simulink model "Proyecto_final_sim_pert_R2020a"  (R2020a)
settings: Solver=VariableStepAuto  StartTime=0.0  StopTime=10.0  RelTol=1e-3
values from neighbouring files (symbols this model uses):
  A = [0 0 1 0 ... (first row only)    [main.m]
  B = [0;0;(Kg*Ki*n_total)/(Rm*(Jb+mb*delta_2^2)*((L/d)));0]    [main.m]
  C = [0 1 0 0]    [main.m]
  D = 0    [main.m]
  L = 0.425    [main.m]    (also in mylqr.m = L'; pole_placement.m = L1)
undefined symbols (not defined in the file or in its folder): K_itae, K_lqr, K_pole, Kext_itae, Kext_lqr, Kext_pole, Kp_itae, Kp_lqr, Kp_pole, rank, sysob_cl_itae, sysob_cl_lqr, sysob_cl_pole, sysob_itae, sysob_lqr, sysob_pole, sysobext_itae, sysobext_lqr, sysobext_pole
settings Model: Creator=Windows_10  LastModifiedBy=sergi

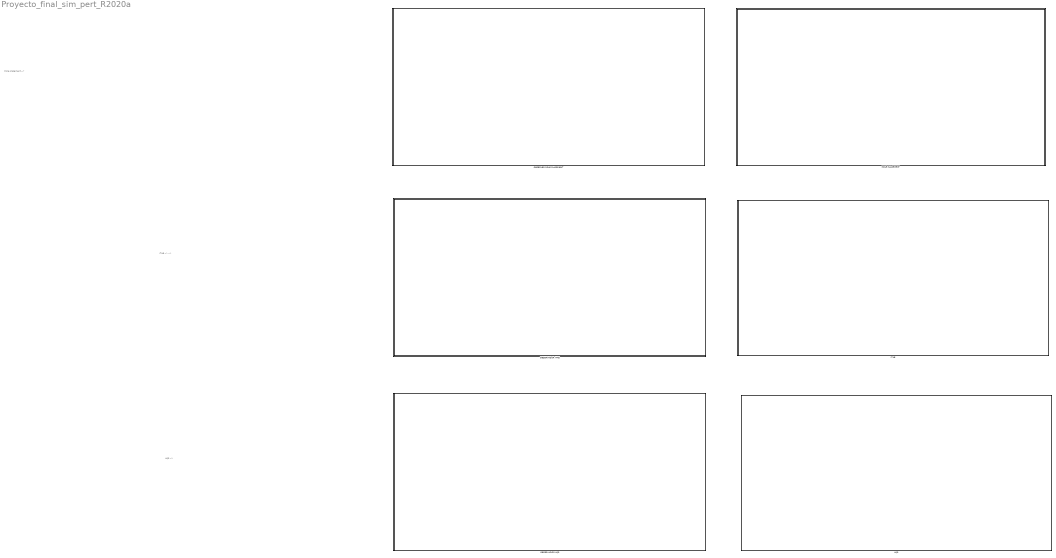
== system Proyecto_final_sim_pert_R2020a ==
  note: LQR -->
  note: ITAE --> -->
  note: Pole placement -->
  ITAE : Subsystem
  LQR : Subsystem
  OBSERVADOR ITAE : Subsystem
  OBSERVADOR LQR : Subsystem
  "OBSERVER POLE PLACEMENT " : Subsystem
  POLE PLACEMENT : Subsystem

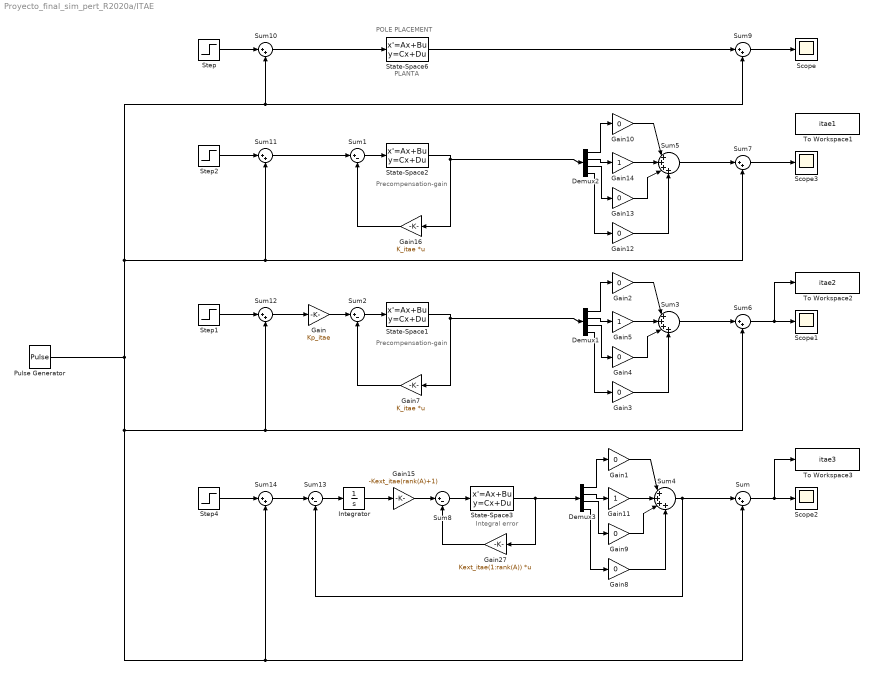
== system Proyecto_final_sim_pert_R2020a/ITAE ==
  note: POLE PLACEMENT
  note: PLANTA
  note: Precompensation-gain
  note: Precompensation-gain
  note: Integral error
  Demux1 : Demux
  Demux2 : Demux
  Demux3 : Demux
  Gain : Gain  Gain=Kp_itae
  Gain{1..4,8..10,12..13} (9 alike) : Gain  Gain=0
  Gain11 : Gain
  Gain14 : Gain
  Gain15 : Gain  Gain=-Kext_itae(rank(A)+1)
  Gain16 : Gain  Gain=K_itae  Multiplication=Matrix(K*u)
  Gain27 : Gain  Gain=Kext_itae(1:rank(A))  Multiplication=Matrix(K*u)
  Gain5 : Gain
  Gain7 : Gain  Gain=K_itae  Multiplication=Matrix(K*u)
  Integrator : Integrator
  Pulse Generator : DiscretePulseGenerator  PulseType=Time based  Period=10  PulseWidth=5
  Scope{,1..3} (4 alike) : Scope
  State-Space{1..3,6} (4 alike) : StateSpace  A=A  B=B  C=eye(rank(A))  D=zeros(rank(A),1)  InitialCondition=0
  Step{,1..2,4} (4 alike) : Step  Time=0  After=L/2  SampleTime=0
  Sum{,6..7,9..12,14} (8 alike) : Sum  Inputs=|++
  Sum{1..2,8,13} (4 alike) : Sum  Inputs=|+-
  Sum3 : Sum  Inputs=|++++
  Sum4 : Sum  Inputs=|++++
  Sum5 : Sum  Inputs=|++++
  To Workspace1 : ToWorkspace  VariableName=itae1  SaveFormat=Timeseries  SampleTime=-1
  To Workspace2 : ToWorkspace  VariableName=itae2  SaveFormat=Timeseries  SampleTime=-1
  To Workspace3 : ToWorkspace  VariableName=itae3  SaveFormat=Timeseries  SampleTime=-1
  wires:
  Sum2/1 -> State-Space1/1
  Gain/1 -> Sum2/1
  Gain7/1 -> Sum2/2
  Gain5/1 -> Sum3/2
  Demux1/1 -> Gain2/1
  Demux1/4 -> Gain3/1
  Gain2/1 -> Sum3/1
  Demux1/3 -> Gain4/1
  Gain4/1 -> Sum3/3
  Demux1/2 -> Gain5/1
  State-Space1/1 -> Demux1/1, Gain7/1
  Gain3/1 -> Sum3/4
  Demux2/3 -> Gain13/1
  Gain10/1 -> Sum5/1
  Demux2/4 -> Gain12/1
  Gain14/1 -> Sum5/2
  Demux2/2 -> Gain14/1
  Gain12/1 -> Sum5/4
  Gain16/1 -> Sum1/2
  State-Space2/1 -> Demux2/1, Gain16/1
  Gain13/1 -> Sum5/3
  Sum1/1 -> State-Space2/1
  Demux2/1 -> Gain10/1
  Gain8/1 -> Sum4/4
  Demux3/3 -> Gain9/1
  Sum8/1 -> State-Space3/1
  Gain1/1 -> Sum4/1
  Gain11/1 -> Sum4/2
  Demux3/2 -> Gain11/1
  Gain9/1 -> Sum4/3
  Demux3/1 -> Gain1/1
  Gain15/1 -> Sum8/1
  Demux3/4 -> Gain8/1
  Sum13/1 -> Integrator/1
  Gain27/1 -> Sum8/2
  Sum4/1 -> Sum/1, Sum13/2
  Integrator/1 -> Gain15/1
  State-Space3/1 -> Gain27/1, Demux3/1
  Sum/1 -> To Workspace3/1, Scope2/1
  Sum3/1 -> Sum6/1
  Sum6/1 -> To Workspace2/1, Scope1/1
  Sum5/1 -> Sum7/1
  Sum7/1 -> Scope3/1
  Sum9/1 -> Scope/1
  State-Space6/1 -> Sum9/1
  Step/1 -> Sum10/1
  Sum10/1 -> State-Space6/1
  Step2/1 -> Sum11/1
  Sum11/1 -> Sum1/1
  Step1/1 -> Sum12/1
  Sum12/1 -> Gain/1
  Sum14/1 -> Sum13/1
  Step4/1 -> Sum14/1
  Pulse Generator/1 -> Sum11/2, Sum7/2, Sum10/2, Sum9/2, Sum6/2, Sum12/2, Sum/2, Sum14/2

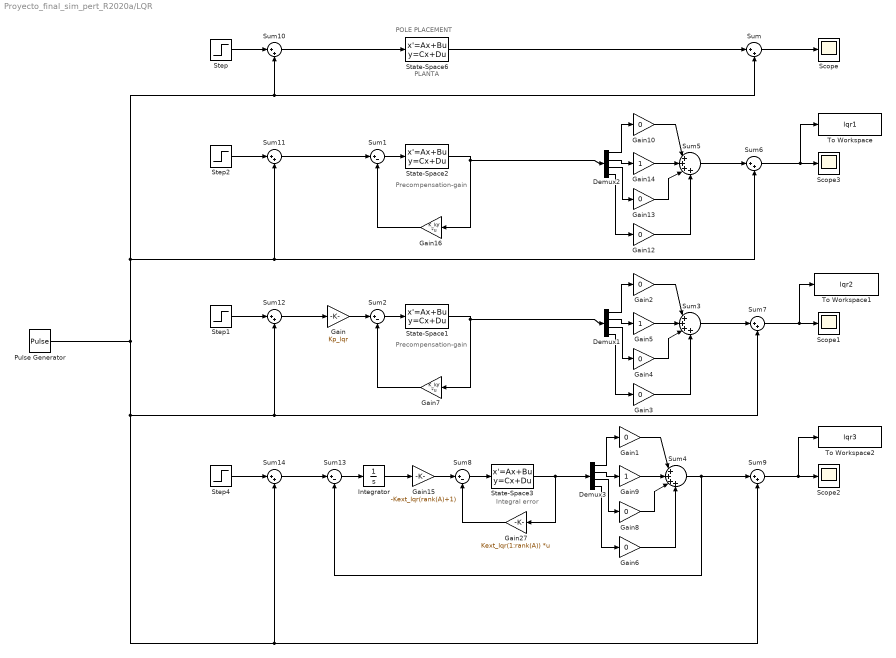
== system Proyecto_final_sim_pert_R2020a/LQR ==
  note: POLE PLACEMENT
  note: PLANTA
  note: Precompensation-gain
  note: Precompensation-gain
  note: Integral error
  Demux1 : Demux
  Demux2 : Demux
  Demux3 : Demux
  Gain : Gain  Gain=Kp_lqr
  Gain{1..4,6,8,10,12..13} (9 alike) : Gain  Gain=0
  Gain14 : Gain
  Gain15 : Gain  Gain=-Kext_lqr(rank(A)+1)
  Gain16 : Gain  Gain=K_lqr  Multiplication=Matrix(K*u)
  Gain27 : Gain  Gain=Kext_lqr(1:rank(A))  Multiplication=Matrix(K*u)
  Gain5 : Gain
  Gain7 : Gain  Gain=K_lqr  Multiplication=Matrix(K*u)
  Gain9 : Gain
  Integrator : Integrator
  Pulse Generator : DiscretePulseGenerator  PulseType=Time based  Period=10  PulseWidth=5
  Scope{,1..3} (4 alike) : Scope
  State-Space{1..3,6} (4 alike) : StateSpace  A=A  B=B  C=eye(rank(A))  D=zeros(rank(A),1)  InitialCondition=0
  Step{,1..2,4} (4 alike) : Step  Time=0  After=L/2  SampleTime=0
  Sum{,6..7,9..12,14} (8 alike) : Sum  Inputs=|++
  Sum{1..2,8,13} (4 alike) : Sum  Inputs=|+-
  Sum3 : Sum  Inputs=|++++
  Sum4 : Sum  Inputs=|++++
  Sum5 : Sum  Inputs=|++++
  To Workspace : ToWorkspace  VariableName=lqr1  SaveFormat=Timeseries  SampleTime=-1
  To Workspace1 : ToWorkspace  VariableName=lqr2  SaveFormat=Timeseries  SampleTime=-1
  To Workspace2 : ToWorkspace  VariableName=lqr3  SaveFormat=Timeseries  SampleTime=-1
  wires:
  Sum2/1 -> State-Space1/1
  Gain/1 -> Sum2/1
  Gain7/1 -> Sum2/2
  Gain5/1 -> Sum3/2
  Demux1/1 -> Gain2/1
  Demux1/4 -> Gain3/1
  Gain2/1 -> Sum3/1
  Demux1/3 -> Gain4/1
  Gain4/1 -> Sum3/3
  Demux1/2 -> Gain5/1
  State-Space1/1 -> Demux1/1, Gain7/1
  Gain3/1 -> Sum3/4
  Demux2/3 -> Gain13/1
  Gain10/1 -> Sum5/1
  Demux2/4 -> Gain12/1
  Gain14/1 -> Sum5/2
  Demux2/2 -> Gain14/1
  Gain12/1 -> Sum5/4
  Gain16/1 -> Sum1/2
  State-Space2/1 -> Demux2/1, Gain16/1
  Gain13/1 -> Sum5/3
  Sum1/1 -> State-Space2/1
  Demux2/1 -> Gain10/1
  Gain15/1 -> Sum8/1
  Sum13/1 -> Integrator/1
  Gain27/1 -> Sum8/2
  State-Space3/1 -> Demux3/1, Gain27/1
  Integrator/1 -> Gain15/1
  Sum8/1 -> State-Space3/1
  Gain6/1 -> Sum4/4
  Gain8/1 -> Sum4/3
  Demux3/3 -> Gain8/1
  Demux3/2 -> Gain9/1
  Demux3/1 -> Gain1/1
  Demux3/4 -> Gain6/1
  Gain1/1 -> Sum4/1
  Gain9/1 -> Sum4/2
  Sum4/1 -> Sum13/2, Sum9/1
  Sum9/1 -> To Workspace2/1, Scope2/1
  Sum7/1 -> To Workspace1/1, Scope1/1
  Sum6/1 -> To Workspace/1, Scope3/1
  Sum5/1 -> Sum6/1
  Sum/1 -> Scope/1
  State-Space6/1 -> Sum/1
  Step/1 -> Sum10/1
  Step2/1 -> Sum11/1
  Step1/1 -> Sum12/1
  Step4/1 -> Sum14/1
  Sum10/1 -> State-Space6/1
  Sum11/1 -> Sum1/1
  Sum12/1 -> Gain/1
  Sum14/1 -> Sum13/1
  Sum3/1 -> Sum7/1
  Pulse Generator/1 -> Sum11/2, Sum6/2, Sum10/2, Sum/2, Sum14/2, Sum9/2, Sum12/2, Sum7/2

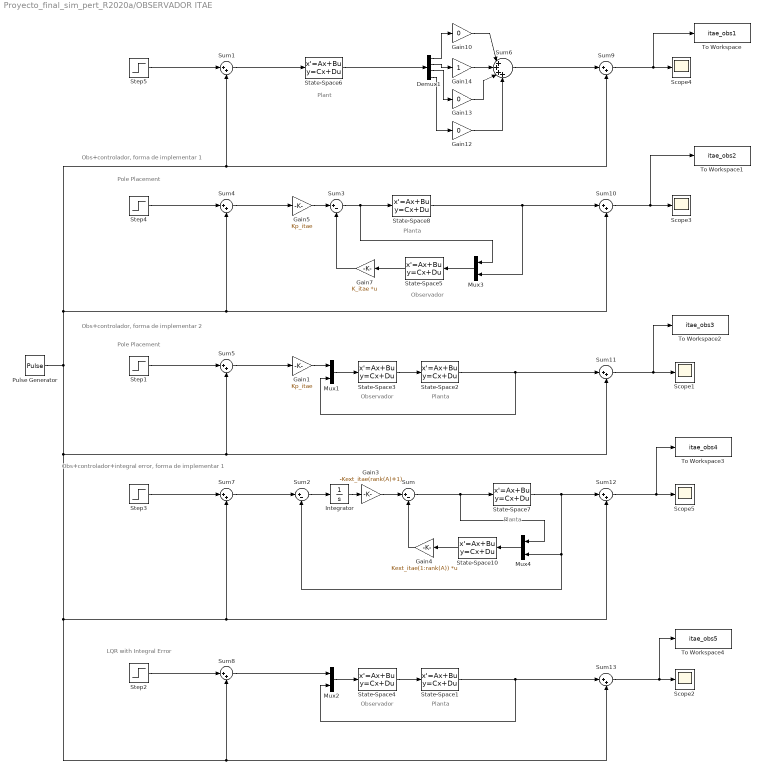
== system Proyecto_final_sim_pert_R2020a/OBSERVADOR ITAE ==
  note: Planta
  note: Planta
  note: Plant
  note: Observador
  note: Pole Placement
  note: Observador
  note: Pole Placement
  note: Obs+controlador, forma de implementar 1
  note: Obs+controlador, forma de implementar 2
  note: Observador
  note: Planta
  note: LQR with Integral Error
  note: Obs+controlador+integral error, forma de implementar 1
  note: Planta
  Demux1 : Demux
  Gain1 : Gain  Gain=Kp_itae
  Gain10 : Gain  Gain=0
  Gain12 : Gain  Gain=0
  Gain13 : Gain  Gain=0
  Gain14 : Gain
  Gain3 : Gain  Gain=-Kext_itae(rank(A)+1)
  Gain4 : Gain  Gain=Kext_itae(1:rank(A))  Multiplication=Matrix(K*u)
  Gain5 : Gain  Gain=Kp_itae
  Gain7 : Gain  Gain=K_itae  Multiplication=Matrix(K*u)
  Integrator : Integrator
  Mux{1..4} (4 alike) : Mux  Inputs=2
  Pulse Generator : DiscretePulseGenerator  PulseType=Time based  Period=10  PulseWidth=5
  Scope{1..5} (5 alike) : Scope
  State-Space{1..2,7..8} (4 alike) : StateSpace  A=A  B=B  C=C  D=D  InitialCondition=0
  State-Space10 : StateSpace  A=sysob_itae.A  B=sysob_itae.B  C=sysob_itae.C  D=sysob_itae.D  InitialCondition=0
  State-Space3 : StateSpace  A=sysob_cl_itae.A  B=sysob_cl_itae.B  C=sysob_cl_itae.C  D=sysob_cl_itae.D  InitialCondition=0
  State-Space4 : StateSpace  A=sysobext_itae.A  B=sysobext_itae.B  C=sysobext_itae.C  D=sysobext_itae.D  InitialCondition=0
  State-Space5 : StateSpace  A=sysob_itae.A  B=sysob_itae.B  C=sysob_itae.C  D=sysob_itae.D  InitialCondition=0
  State-Space6 : StateSpace  A=A  B=B  C=eye(rank(A))  D=zeros(rank(A),1)  InitialCondition=0
  Step{1..5} (5 alike) : Step  Time=0  After=L/2  SampleTime=0
  Sum : Sum  Inputs=|+-
  Sum{1,4..5,7..13} (10 alike) : Sum  Inputs=|++
  Sum2 : Sum  Inputs=|+-
  Sum3 : Sum  Inputs=|+-
  Sum6 : Sum  Inputs=|++++
  To Workspace : ToWorkspace  VariableName=itae_obs1  SaveFormat=Timeseries  SampleTime=-1
  To Workspace1 : ToWorkspace  VariableName=itae_obs2  SaveFormat=Timeseries  SampleTime=-1
  To Workspace2 : ToWorkspace  VariableName=itae_obs3  SaveFormat=Timeseries  SampleTime=-1
  To Workspace3 : ToWorkspace  VariableName=itae_obs4  SaveFormat=Timeseries  SampleTime=-1
  To Workspace4 : ToWorkspace  VariableName=itae_obs5  SaveFormat=Timeseries  SampleTime=-1
  wires:
  Gain7/1 -> Sum3/2
  State-Space2/1 -> Mux1/2, Sum11/1
  Demux1/2 -> Gain14/1
  State-Space3/1 -> State-Space2/1
  Demux1/3 -> Gain13/1
  Gain1/1 -> Mux1/1
  Gain13/1 -> Sum6/3
  Mux1/1 -> State-Space3/1
  State-Space5/1 -> Gain7/1
  Gain5/1 -> Sum3/1
  Mux3/1 -> State-Space5/1
  Sum3/1 -> Mux3/1, State-Space8/1
  State-Space8/1 -> Sum10/1, Mux3/2
  Demux1/1 -> Gain10/1
  State-Space6/1 -> Demux1/1
  Gain10/1 -> Sum6/1
  Gain14/1 -> Sum6/2
  Demux1/4 -> Gain12/1
  Gain12/1 -> Sum6/4
  Mux2/1 -> State-Space4/1
  State-Space1/1 -> Sum13/1, Mux2/2
  State-Space4/1 -> State-Space1/1
  Integrator/1 -> Gain3/1
  Gain3/1 -> Sum/1
  Mux4/1 -> State-Space10/1
  State-Space10/1 -> Gain4/1
  Sum2/1 -> Integrator/1
  Sum/1 -> State-Space7/1, Mux4/1
  Gain4/1 -> Sum/2
  State-Space7/1 -> Sum12/1, Sum2/2, Mux4/2
  Step5/1 -> Sum1/1
  Sum1/1 -> State-Space6/1
  Step4/1 -> Sum4/1
  Sum4/1 -> Gain5/1
  Step1/1 -> Sum5/1
  Sum5/1 -> Gain1/1
  Step3/1 -> Sum7/1
  Sum7/1 -> Sum2/1
  Step2/1 -> Sum8/1
  Sum8/1 -> Mux2/1
  Sum6/1 -> Sum9/1
  Sum9/1 -> To Workspace/1, Scope4/1
  Sum10/1 -> To Workspace1/1, Scope3/1
  Sum11/1 -> To Workspace2/1, Scope1/1
  Sum12/1 -> To Workspace3/1, Scope5/1
  Sum13/1 -> To Workspace4/1, Scope2/1
  Pulse Generator/1 -> Sum4/2, Sum10/2, Sum1/2, Sum9/2, Sum5/2, Sum11/2, Sum7/2, Sum12/2, Sum8/2, Sum13/2

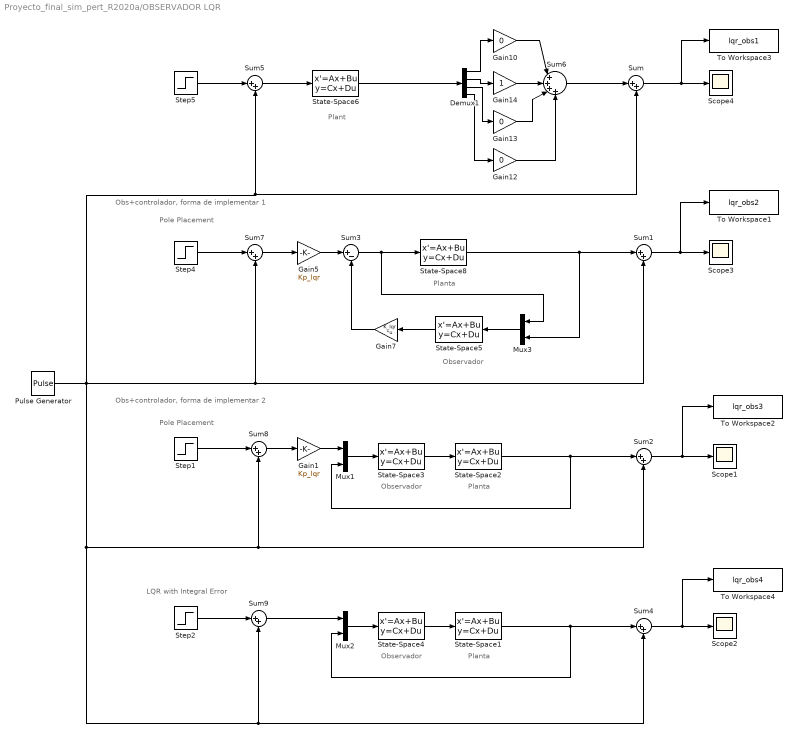
== system Proyecto_final_sim_pert_R2020a/OBSERVADOR LQR ==
  note: Planta
  note: Planta
  note: Plant
  note: Observador
  note: Pole Placement
  note: Observador
  note: Pole Placement
  note: Obs+controlador, forma de implementar 1
  note: Obs+controlador, forma de implementar 2
  note: Observador
  note: Planta
  note: LQR with Integral Error
  Demux1 : Demux
  Gain1 : Gain  Gain=Kp_lqr
  Gain10 : Gain  Gain=0
  Gain12 : Gain  Gain=0
  Gain13 : Gain  Gain=0
  Gain14 : Gain
  Gain5 : Gain  Gain=Kp_lqr
  Gain7 : Gain  Gain=K_lqr  Multiplication=Matrix(K*u)
  Mux1 : Mux  Inputs=2
  Mux2 : Mux  Inputs=2
  Mux3 : Mux  Inputs=2
  Pulse Generator : DiscretePulseGenerator  PulseType=Time based  Period=10  PulseWidth=5
  Scope{1..4} (4 alike) : Scope
  State-Space1 : StateSpace  A=A  B=B  C=C  D=D  InitialCondition=0
  State-Space2 : StateSpace  A=A  B=B  C=C  D=D  InitialCondition=0
  State-Space3 : StateSpace  A=sysob_cl_lqr.A  B=sysob_cl_lqr.B  C=sysob_cl_lqr.C  D=sysob_cl_lqr.D  InitialCondition=0
  State-Space4 : StateSpace  A=sysobext_lqr.A  B=sysobext_lqr.B  C=sysobext_lqr.C  D=sysobext_lqr.D  InitialCondition=0
  State-Space5 : StateSpace  A=sysob_lqr.A  B=sysob_lqr.B  C=sysob_lqr.C  D=sysob_lqr.D  InitialCondition=0
  State-Space6 : StateSpace  A=A  B=B  C=eye(rank(A))  D=zeros(rank(A),1)  InitialCondition=0
  State-Space8 : StateSpace  A=A  B=B  C=C  D=D  InitialCondition=0
  Step{1..2,4..5} (4 alike) : Step  Time=0  After=L/2  SampleTime=0
  Sum{,1..2,4..5,7..9} (8 alike) : Sum  Inputs=|++
  Sum3 : Sum  Inputs=|+-
  Sum6 : Sum  Inputs=|++++
  To Workspace1 : ToWorkspace  VariableName=lqr_obs2  SaveFormat=Timeseries  SampleTime=-1
  To Workspace2 : ToWorkspace  VariableName=lqr_obs3  SaveFormat=Timeseries  SampleTime=-1
  To Workspace3 : ToWorkspace  VariableName=lqr_obs1  SaveFormat=Timeseries  SampleTime=-1
  To Workspace4 : ToWorkspace  VariableName=lqr_obs4  SaveFormat=Timeseries  SampleTime=-1
  wires:
  Gain7/1 -> Sum3/2
  State-Space2/1 -> Sum2/1, Mux1/2
  Demux1/2 -> Gain14/1
  State-Space3/1 -> State-Space2/1
  Demux1/3 -> Gain13/1
  Gain1/1 -> Mux1/1
  Gain13/1 -> Sum6/3
  Mux1/1 -> State-Space3/1
  State-Space5/1 -> Gain7/1
  Gain5/1 -> Sum3/1
  Mux3/1 -> State-Space5/1
  Sum3/1 -> Mux3/1, State-Space8/1
  State-Space8/1 -> Sum1/1, Mux3/2
  Demux1/1 -> Gain10/1
  State-Space6/1 -> Demux1/1
  Gain10/1 -> Sum6/1
  Gain14/1 -> Sum6/2
  Demux1/4 -> Gain12/1
  Gain12/1 -> Sum6/4
  Mux2/1 -> State-Space4/1
  State-Space1/1 -> Sum4/1, Mux2/2
  State-Space4/1 -> State-Space1/1
  Sum6/1 -> Sum/1
  Sum/1 -> To Workspace3/1, Scope4/1
  Sum1/1 -> Scope3/1, To Workspace1/1
  Sum2/1 -> Scope1/1, To Workspace2/1
  Sum4/1 -> Scope2/1, To Workspace4/1
  Sum5/1 -> State-Space6/1
  Step5/1 -> Sum5/1
  Sum7/1 -> Gain5/1
  Step4/1 -> Sum7/1
  Sum8/1 -> Gain1/1
  Step1/1 -> Sum8/1
  Sum9/1 -> Mux2/1
  Step2/1 -> Sum9/1
  Pulse Generator/1 -> Sum1/2, Sum7/2, Sum8/2, Sum2/2, Sum4/2, Sum9/2, Sum/2, Sum5/2

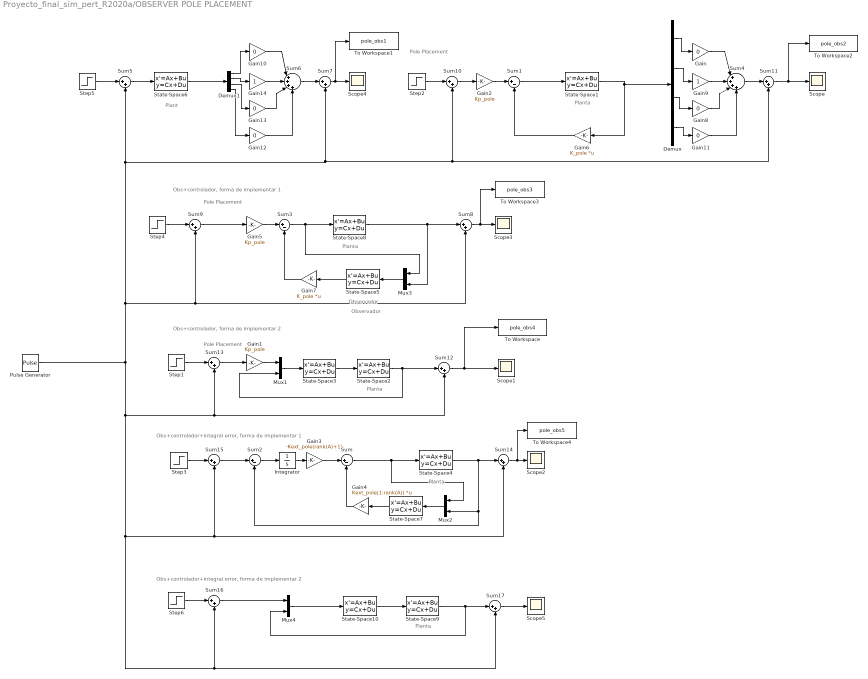
== system Proyecto_final_sim_pert_R2020a/OBSERVER POLE PLACEMENT  ==
  note: Planta
  note: Planta
  note: Planta
  note: Planta
  note: Planta
  note: Plant
  note: Obs+controlador+integral error, forma de implementar 1
  note: Observador
  note: Pole Placement
  note: Pole Placement
  note: Observador
  note: Pole Placement
  note: Obs+controlador, forma de implementar 1
  note: Obs+controlador, forma de implementar 2
  note: Obs+controlador+integral error, forma de implementar 2
  Demux : Demux
  Demux1 : Demux
  Gain{,8,10..13} (6 alike) : Gain  Gain=0
  Gain1 : Gain  Gain=Kp_pole
  Gain14 : Gain
  Gain2 : Gain  Gain=Kp_pole
  Gain3 : Gain  Gain=-Kext_pole(rank(A)+1)
  Gain4 : Gain  Gain=Kext_pole(1:rank(A))  Multiplication=Matrix(K*u)
  Gain5 : Gain  Gain=Kp_pole
  Gain6 : Gain  Gain=K_pole  Multiplication=Matrix(K*u)
  Gain7 : Gain  Gain=K_pole  Multiplication=Matrix(K*u)
  Gain9 : Gain
  Integrator : Integrator
  Mux{1..4} (4 alike) : Mux  Inputs=2
  Pulse Generator : DiscretePulseGenerator  PulseType=Time based  Period=10  PulseWidth=5
  Scope{,1..5} (6 alike) : Scope
  State-Space1 : StateSpace  A=A  B=B  C=eye(rank(A))  D=zeros(rank(A),1)  InitialCondition=0
  State-Space10 : StateSpace  A=sysobext_pole.A  B=sysobext_pole.B  C=sysobext_pole.C  D=sysobext_pole.D  InitialCondition=0
  State-Space{2,4,8..9} (4 alike) : StateSpace  A=A  B=B  C=C  D=D  InitialCondition=0
  State-Space3 : StateSpace  A=sysob_cl_pole.A  B=sysob_cl_pole.B  C=sysob_cl_pole.C  D=sysob_cl_pole.D  InitialCondition=0
  State-Space5 : StateSpace  A=sysob_pole.A  B=sysob_pole.B  C=sysob_pole.C  D=sysob_pole.D  InitialCondition=0
  State-Space6 : StateSpace  A=A  B=B  C=eye(rank(A))  D=zeros(rank(A),1)  InitialCondition=0
  State-Space7 : StateSpace  A=sysob_pole.A  B=sysob_pole.B  C=sysob_pole.C  D=sysob_pole.D  InitialCondition=0
  Step{1..6} (6 alike) : Step  Time=0  After=L/2  SampleTime=0
  Sum{,1..3} (4 alike) : Sum  Inputs=|+-
  Sum{5,7..17} (12 alike) : Sum  Inputs=|++
  Sum4 : Sum  Inputs=|++++
  Sum6 : Sum  Inputs=|++++
  To Workspace : ToWorkspace  VariableName=pole_obs4  SaveFormat=Timeseries  SampleTime=-1
  To Workspace1 : ToWorkspace  VariableName=pole_obs1  SaveFormat=Timeseries  SampleTime=-1
  To Workspace2 : ToWorkspace  VariableName=pole_obs2  SaveFormat=Timeseries  SampleTime=-1
  To Workspace3 : ToWorkspace  VariableName=pole_obs3  SaveFormat=Timeseries  SampleTime=-1
  To Workspace4 : ToWorkspace  VariableName=pole_obs5  SaveFormat=Timeseries  SampleTime=-1
  wires:
  Gain4/1 -> Sum/2
  Gain7/1 -> Sum3/2
  Gain6/1 -> Sum1/2
  Sum/1 -> State-Space4/1, Mux2/1
  Demux1/2 -> Gain14/1
  State-Space3/1 -> State-Space2/1
  Demux1/3 -> Gain13/1
  Demux/2 -> Gain9/1
  Gain1/1 -> Mux1/1
  Gain13/1 -> Sum6/3
  Mux1/1 -> State-Space3/1
  State-Space5/1 -> Gain7/1
  Gain5/1 -> Sum3/1
  Sum1/1 -> State-Space1/1
  State-Space4/1 -> Sum14/1, Sum2/2, Mux2/2
  Mux3/1 -> State-Space5/1
  Sum3/1 -> Mux3/1, State-Space8/1
  Gain2/1 -> Sum1/1
  State-Space8/1 -> Sum8/1, Mux3/2
  Mux4/1 -> State-Space10/1
  Demux/1 -> Gain/1
  Mux2/1 -> State-Space7/1
  State-Space7/1 -> Gain4/1
  Gain/1 -> Sum4/1
  Demux1/1 -> Gain10/1
  Sum2/1 -> Integrator/1
  State-Space6/1 -> Demux1/1
  Gain10/1 -> Sum6/1
  Gain3/1 -> Sum/1
  Integrator/1 -> Gain3/1
  State-Space1/1 -> Demux/1, Gain6/1
  State-Space9/1 -> Sum17/1, Mux4/2
  Gain8/1 -> Sum4/3
  Gain14/1 -> Sum6/2
  Gain9/1 -> Sum4/2
  Demux/3 -> Gain8/1
  State-Space10/1 -> State-Space9/1
  Demux/4 -> Gain11/1
  Gain11/1 -> Sum4/4
  Demux1/4 -> Gain12/1
  Gain12/1 -> Sum6/4
  Step5/1 -> Sum5/1
  Sum6/1 -> Sum7/1
  Sum7/1 -> To Workspace1/1, Scope4/1
  Sum8/1 -> To Workspace3/1, Scope3/1
  Sum5/1 -> State-Space6/1
  Pulse Generator/1 -> Sum10/2, Sum11/2, Sum7/2, Sum5/2, Sum9/2, Sum8/2, Sum12/2, Sum13/2, Sum17/2, Sum16/2, Sum15/2, Sum14/2
  Step4/1 -> Sum9/1
  Sum9/1 -> Gain5/1
  Sum4/1 -> Sum11/1
  Sum11/1 -> To Workspace2/1, Scope/1
  Step2/1 -> Sum10/1
  Sum10/1 -> Gain2/1
  Sum12/1 -> To Workspace/1, Scope1/1
  Sum13/1 -> Gain1/1
  Step1/1 -> Sum13/1
  State-Space2/1 -> Sum12/1, Mux1/2
  Sum14/1 -> To Workspace4/1, Scope2/1
  Sum15/1 -> Sum2/1
  Step3/1 -> Sum15/1
  Step6/1 -> Sum16/1
  Sum16/1 -> Mux4/1
  Sum17/1 -> Scope5/1

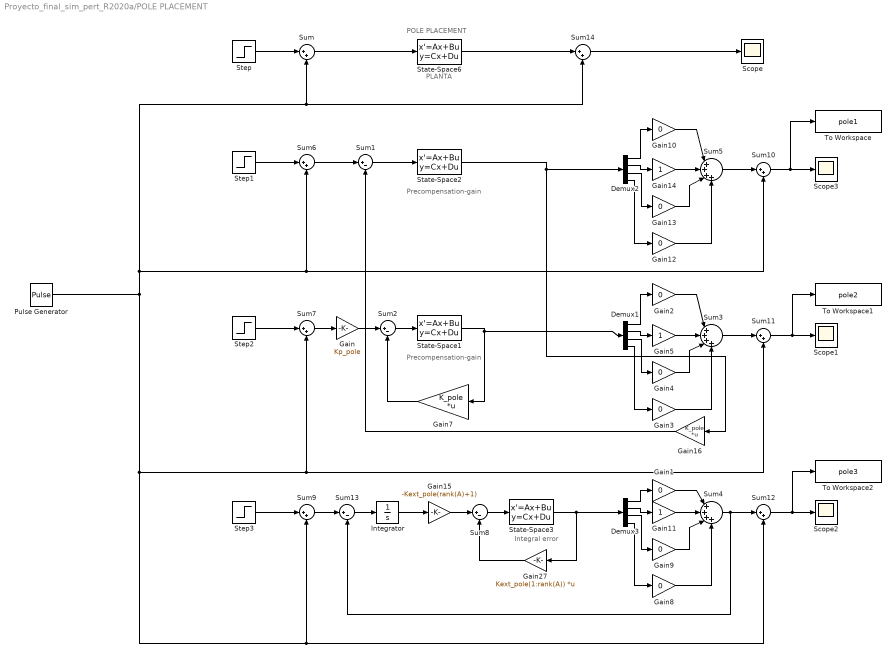
== system Proyecto_final_sim_pert_R2020a/POLE PLACEMENT ==
  note: POLE PLACEMENT
  note: PLANTA
  note: Precompensation-gain
  note: Integral error
  note: Precompensation-gain
  Demux1 : Demux
  Demux2 : Demux
  Demux3 : Demux
  Gain : Gain  Gain=Kp_pole
  Gain{1..4,8..10,12..13} (9 alike) : Gain  Gain=0
  Gain11 : Gain
  Gain14 : Gain
  Gain15 : Gain  Gain=-Kext_pole(rank(A)+1)
  Gain16 : Gain  Gain=K_pole  Multiplication=Matrix(K*u)
  Gain27 : Gain  Gain=Kext_pole(1:rank(A))  Multiplication=Matrix(K*u)
  Gain5 : Gain
  Gain7 : Gain  Gain=K_pole  Multiplication=Matrix(K*u)
  Integrator : Integrator
  Pulse Generator : DiscretePulseGenerator  PulseType=Time based  Period=10  PulseWidth=5
  Scope{,1..3} (4 alike) : Scope
  State-Space1 : StateSpace  A=A  B=B  C=eye(rank(A))  D=zeros(rank(A),1)  InitialCondition=0
  State-Space2 : StateSpace  A=A  B=B  C=eye(rank(A))  D=zeros(rank(A),1)  InitialCondition=0
  State-Space3 : StateSpace  A=A  B=B  C=eye(rank(A))  D=zeros(rank(A),1)  InitialCondition=0
  State-Space6 : StateSpace  A=A  B=B  C=C  D=D  InitialCondition=0
  Step{,1..3} (4 alike) : Step  Time=0  After=L/2  SampleTime=0
  Sum{,6..7,9..12,14} (8 alike) : Sum  Inputs=|++
  Sum{1..2,8,13} (4 alike) : Sum  Inputs=|+-
  Sum3 : Sum  Inputs=|++++
  Sum4 : Sum  Inputs=|++++
  Sum5 : Sum  Inputs=|++++
  To Workspace : ToWorkspace  VariableName=pole1  SaveFormat=Timeseries  SampleTime=-1
  To Workspace1 : ToWorkspace  VariableName=pole2  SaveFormat=Timeseries  SampleTime=-1
  To Workspace2 : ToWorkspace  VariableName=pole3  SaveFormat=Timeseries  SampleTime=-1
  wires:
  Gain27/1 -> Sum8/2
  Sum13/1 -> Integrator/1
  Gain15/1 -> Sum8/1
  Sum2/1 -> State-Space1/1
  Sum8/1 -> State-Space3/1
  Gain/1 -> Sum2/1
  Gain7/1 -> Sum2/2
  Integrator/1 -> Gain15/1
  Gain5/1 -> Sum3/2
  Demux1/1 -> Gain2/1
  Demux1/4 -> Gain3/1
  Gain2/1 -> Sum3/1
  Demux1/3 -> Gain4/1
  Gain4/1 -> Sum3/3
  Demux1/2 -> Gain5/1
  State-Space1/1 -> Demux1/1, Gain7/1
  Gain3/1 -> Sum3/4
  State-Space3/1 -> Gain27/1, Demux3/1
  Demux3/3 -> Gain9/1
  Demux3/4 -> Gain8/1
  Demux3/1 -> Gain1/1
  Sum4/1 -> Sum12/1, Sum13/2
  Gain8/1 -> Sum4/4
  Gain9/1 -> Sum4/3
  Gain11/1 -> Sum4/2
  Gain1/1 -> Sum4/1
  Demux3/2 -> Gain11/1
  Demux2/3 -> Gain13/1
  Gain10/1 -> Sum5/1
  Demux2/4 -> Gain12/1
  Gain14/1 -> Sum5/2
  Demux2/2 -> Gain14/1
  Gain12/1 -> Sum5/4
  Gain16/1 -> Sum1/2
  State-Space2/1 -> Demux2/1, Gain16/1
  Gain13/1 -> Sum5/3
  Sum1/1 -> State-Space2/1
  Demux2/1 -> Gain10/1
  Step/1 -> Sum/1
  Step1/1 -> Sum6/1
  Step2/1 -> Sum7/1
  Step3/1 -> Sum9/1
  Sum/1 -> State-Space6/1
  Sum6/1 -> Sum1/1
  Sum7/1 -> Gain/1
  Sum9/1 -> Sum13/1
  Sum5/1 -> Sum10/1
  Sum10/1 -> To Workspace/1, Scope3/1
  Sum3/1 -> Sum11/1
  Sum11/1 -> Scope1/1, To Workspace1/1
  Sum12/1 -> To Workspace2/1, Scope2/1
  State-Space6/1 -> Sum14/1
  Sum14/1 -> Scope/1
  Pulse Generator/1 -> Sum11/2, Sum7/2, Sum9/2, Sum12/2, Sum14/2, Sum/2, Sum6/2, Sum10/2
